simulink model "Doppelpendel_LQG_2016a"  (R2016a)
settings: Solver=ode45  StartTime=0.0  StopTime=10
values from neighbouring files (symbols this model uses):
  Beobachter_Rueckfuehrung = 0    [m8.m]
  parLQR = LQR_Entwurf( sysd,parLQR )    [m8.m]
  Quantisierung = 0    [m8.m]
undefined symbols (not defined in the file or in its folder): parDP, parKAL
libraries: cstblocks x3
settings Model: Creator=tg  LastModifiedBy=Meiner
settings DataIOCC: LimitDataPoints=on  SaveFormat=Array  SignalLoggingSaveFormat=ModelDataLogs
settings OptimizationCC: ExpressionDepthLimit=2147483647  InitFltsAndDblsToZero=on
settings DebuggingCC: UnderspecifiedInitializationDetection=Classic  MergeDetectMultiDrivingBlocksExec=none  SolverPrmCheckMsg=warning  FcnCallInpInsideContextMsg=EnableAllAsWarning  StateNameClashWarn=warning
settings HardwareCC: ProdBitPerPointer=32  ProdLargestAtomicFloat=None  ProdIntDivRoundTo=Undefined  ProdEndianess=Unspecified  ProdWordSize=32  ProdHWDeviceType=32-bit Generic
settings ModelReferenceCC: PropagateSignalLabelsOutOfModel=off
settings SFSimCC: SimParseCustomCode=off
settings GRTTargetCC: CombineOutputUpdateFcns=off  GRTInterface=on

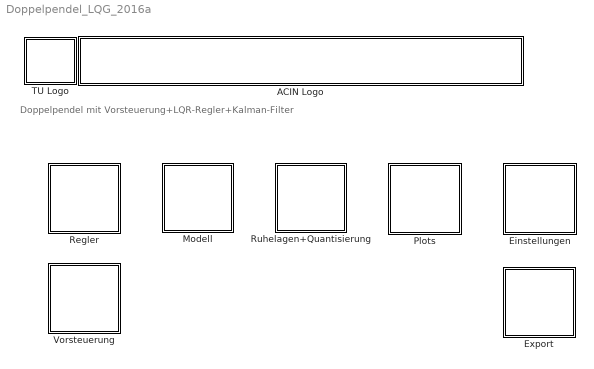
== system Doppelpendel_LQG_2016a ==
  note: Doppelpendel mit Vorsteuerung+LQR-Regler+Kalman-Filter
  ACIN Logo : Subsystem
      mask init:
      | s = get_param(gcb,'UserData');
      mask Display:
      | image(s.logo,[0 0 439 45]);
      | %axis image
  Einstellungen : Subsystem
  Export : Subsystem
  Modell : Subsystem
  Plots : Subsystem
  Regler : Subsystem
  Ruhelagen+Quantisierung : Subsystem
  TU Logo : Subsystem
      mask init:
      | s = get_param(gcb,'UserData');
      mask Display: image(s.logo,[0 0 45 45]);
  Vorsteuerung : Subsystem

== system Doppelpendel_LQG_2016a/ACIN Logo ==

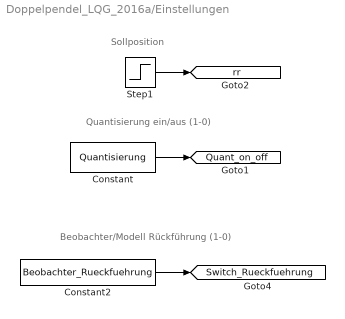
== system Doppelpendel_LQG_2016a/Einstellungen ==
  note: Sollposition
  note: Quantisierung ein/aus (1-0)
  note: Beobachter/Modell Rückführung (1-0)
  Constant : Constant  Value=Quantisierung
  Constant2 : Constant  Value=Beobachter_Rueckfuehrung
  Step1 : Step  After=0.1  SampleTime=parLQR.Ta
  tag scope: Quant_on_off=global, Switch_Rueckfuehrung=global, rr=global
  wires:
  Step1/1 -> [rr]
  Constant/1 -> [Quant_on_off]
  Constant2/1 -> [Switch_Rueckfuehrung]

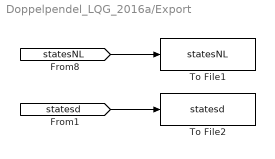
== system Doppelpendel_LQG_2016a/Export ==
  To File1 : ToFile  Filename=statesNL  MatrixName=data  SampleTime=parDP.Ta
  To File2 : ToFile  Filename=statesd  MatrixName=data  SampleTime=parDP.Ta
  wires:
  [statesNL] -> To File1/1
  [statesd] -> To File2/1

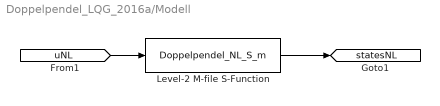
== system Doppelpendel_LQG_2016a/Modell ==
  Level-2 M-file S-Function : M-S-Function  FunctionName=Doppelpendel_NL_S_m  Parameters=parDP.phi10,parDP.omega10,parDP.phi20,parDP.omega20,parDP.s0,parDP.w0,parDP.l1,parDP.l2,parDP.a1,parDP.a2,parDP.m1,parDP.m2,parDP.J1,parDP.J2,parDP.d1,parDP.d2
  tag scope: statesNL=global
  wires:
  [uNL] -> Level-2 M-file S-Function/1
  Level-2 M-file S-Function/1 -> [statesNL]

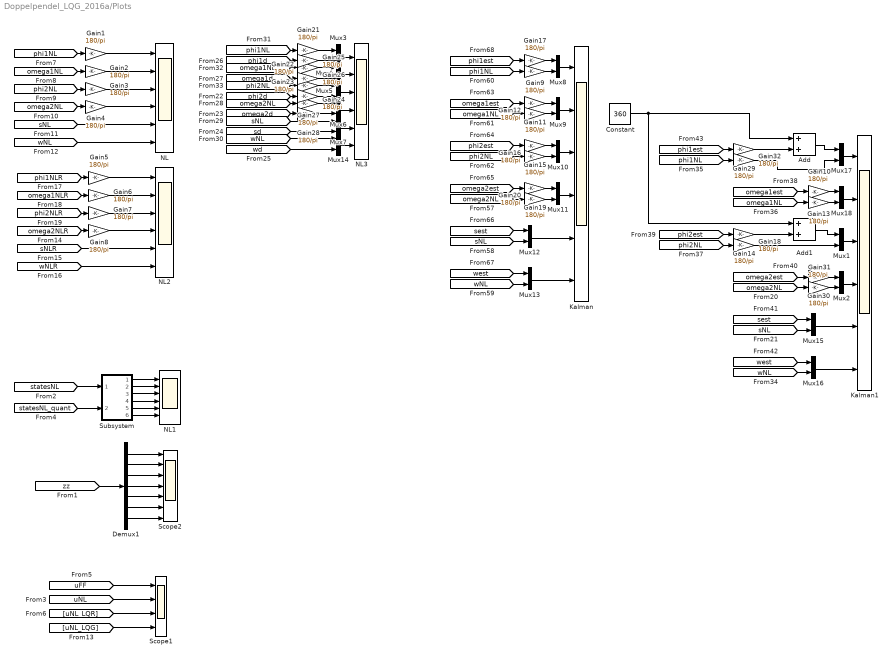
== system Doppelpendel_LQG_2016a/Plots ==
  Add : Sum
  Add1 : Sum
  Constant : Constant  Value=360
  Demux1 : Demux  Outputs=7
  Gain{1..32} (32 alike) : Gain  Gain=180/pi
  Kalman : Scope  NumInputPorts=6
  Kalman1 : Scope  NumInputPorts=6
  Mux{1..18} (18 alike) : Mux  Inputs=2
  NL{,1..3} (4 alike) : Scope  NumInputPorts=6
  Scope1 : Scope  NumInputPorts=4
  Scope2 : Scope  NumInputPorts=7
  Subsystem : Subsystem
  wires:
  [omega1NL] -> Gain2/1
  [omega2NL] -> Gain4/1
  [sNL] -> NL/5
  [wNL] -> NL/6
  Gain1/1 -> NL/1
  Gain2/1 -> NL/2
  Gain3/1 -> NL/3
  Gain4/1 -> NL/4
  [phi1NL] -> Gain1/1
  [phi2NL] -> Gain3/1
  [statesNL] -> Subsystem/1(In1)
  [statesNL_quant] -> Subsystem/2(In2)
  Subsystem/1(Out1) -> NL1/1
  Subsystem/2(Out2) -> NL1/2
  Subsystem/3(Out3) -> NL1/3
  Subsystem/4(Out4) -> NL1/4
  Subsystem/5(Out5) -> NL1/5
  Subsystem/6(Out6) -> NL1/6
  [omega1NL] -> Gain22/1
  [omega2NL] -> Gain24/1
  [phi1NL] -> Gain21/1
  [phi2NL] -> Gain23/1
  Mux3/1 -> NL3/1
  Mux4/1 -> NL3/2
  Mux5/1 -> NL3/3
  Mux6/1 -> NL3/4
  Mux7/1 -> NL3/5
  Mux14/1 -> NL3/6
  Gain21/1 -> Mux3/1
  Gain22/1 -> Mux4/1
  Gain23/1 -> Mux5/1
  Gain24/1 -> Mux6/1
  [sNL] -> Mux7/1
  [wNL] -> Mux14/1
  [phi1d] -> Gain25/1
  [omega1d] -> Gain26/1
  [phi2d] -> Gain27/1
  [omega2d] -> Gain28/1
  Gain25/1 -> Mux3/2
  Gain26/1 -> Mux4/2
  Gain27/1 -> Mux5/2
  Gain28/1 -> Mux6/2
  [sd] -> Mux7/2
  [wd] -> Mux14/2
  Demux1/1 -> Scope2/1
  Demux1/2 -> Scope2/2
  Demux1/3 -> Scope2/3
  Demux1/4 -> Scope2/4
  Demux1/5 -> Scope2/5
  Demux1/6 -> Scope2/6
  Demux1/7 -> Scope2/7
  [zz] -> Demux1/1
  Mux13/1 -> Kalman/6
  Mux12/1 -> Kalman/5
  Mux11/1 -> Kalman/4
  [omega1NL] -> Gain12/1
  [omega2NL] -> Gain20/1
  [phi1NL] -> Gain9/1
  [phi2NL] -> Gain16/1
  [sest] -> Mux12/1
  [west] -> Mux13/1
  [sNL] -> Mux12/2
  [wNL] -> Mux13/2
  Gain9/1 -> Mux8/2
  Gain17/1 -> Mux8/1
  [phi1est] -> Gain17/1
  Mux8/1 -> Kalman/1
  Gain12/1 -> Mux9/2
  Gain11/1 -> Mux9/1
  Mux9/1 -> Kalman/2
  [omega1est] -> Gain11/1
  Gain16/1 -> Mux10/2
  Gain15/1 -> Mux10/1
  [phi2est] -> Gain15/1
  Mux10/1 -> Kalman/3
  Gain20/1 -> Mux11/2
  Gain19/1 -> Mux11/1
  [omega2est] -> Gain19/1
  [uFF] -> Scope1/1
  [uNL] -> Scope1/2
  [uNL_LQR] -> Scope1/3
  [uNL_LQG] -> Scope1/4
  [omega1NLR] -> Gain6/1
  [omega2NLR] -> Gain8/1
  [sNLR] -> NL2/5
  [wNLR] -> NL2/6
  Gain5/1 -> NL2/1
  Gain6/1 -> NL2/2
  Gain7/1 -> NL2/3
  Gain8/1 -> NL2/4
  [phi1NLR] -> Gain5/1
  [phi2NLR] -> Gain7/1
  Mux16/1 -> Kalman1/6
  Mux15/1 -> Kalman1/5
  Mux2/1 -> Kalman1/4
  [omega1NL] -> Gain13/1
  [omega2NL] -> Gain31/1
  [phi1NL] -> Gain32/1
  [phi2NL] -> Gain18/1
  [sest] -> Mux15/1
  [west] -> Mux16/1
  [sNL] -> Mux15/2
  [wNL] -> Mux16/2
  Gain32/1 -> Mux17/2
  Gain29/1 -> Add/2
  [phi1est] -> Gain29/1
  Mux17/1 -> Kalman1/1
  Gain13/1 -> Mux18/2
  Gain10/1 -> Mux18/1
  Mux18/1 -> Kalman1/2
  [omega1est] -> Gain10/1
  Gain18/1 -> Mux1/2
  Gain14/1 -> Add1/2
  [phi2est] -> Gain14/1
  Mux1/1 -> Kalman1/3
  Gain31/1 -> Mux2/2
  Gain30/1 -> Mux2/1
  [omega2est] -> Gain30/1
  Add/1 -> Mux17/1
  Constant/1 -> Add/1, Add1/1
  Add1/1 -> Mux1/1

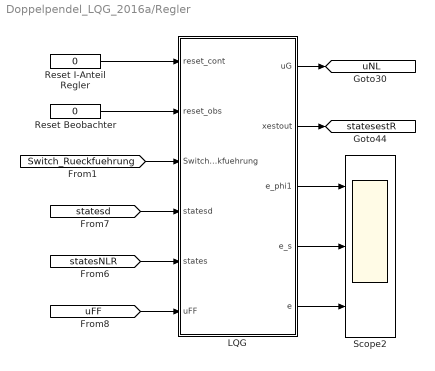
== system Doppelpendel_LQG_2016a/Regler ==
  LQG : MATLAB Function  TreatAsAtomicUnit=on
      settings: PermitHierarchicalResolution=ParametersOnly
  Reset Beobachter : Constant  Value=0
  Reset I-Anteil Regler : Constant  Value=0
  Scope2 : Scope  NumInputPorts=3
  tag scope: statesestR=global, uNL=global
  wires:
  LQG/3(e_phi1) -> Scope2/1
  LQG/4(e_s) -> Scope2/2
  LQG/5(e) -> Scope2/3
  [statesNLR] -> LQG/5(states)
  LQG/2(xestout) -> [statesestR]
  [statesd] -> LQG/4(statesd)
  [uFF] -> LQG/6(uFF)
  LQG/1(uG) -> [uNL]
  Reset Beobachter/1 -> LQG/2(reset_obs)
  Reset I-Anteil Regler/1 -> LQG/1(reset_cont)
  [Switch_Rueckfuehrung] -> LQG/3(Switch_Rueckfuehrung)

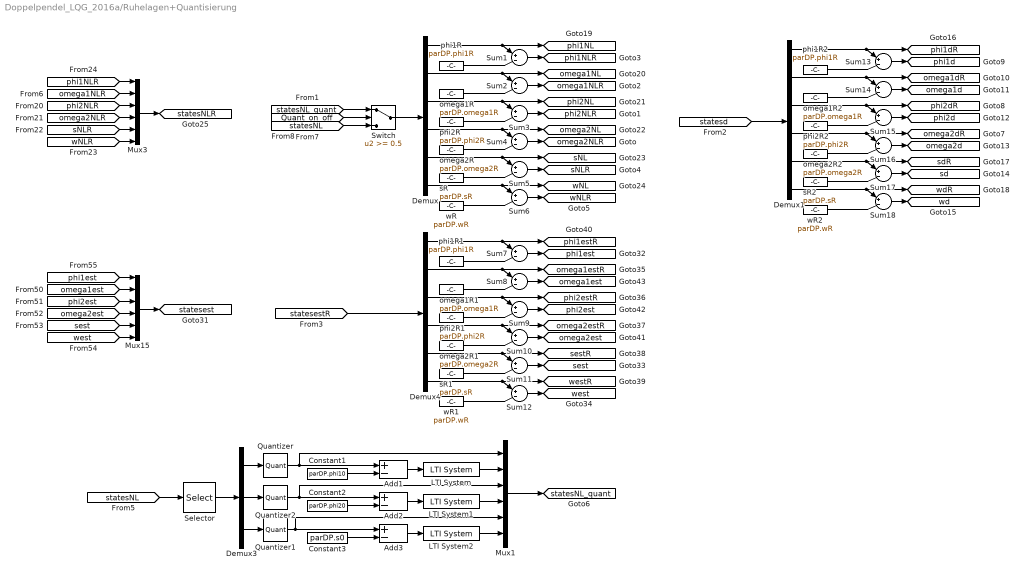
== system Doppelpendel_LQG_2016a/Ruhelagen+Quantisierung ==
  Add1 : Sum  Inputs=+-
  Add2 : Sum  Inputs=+-
  Add3 : Sum  Inputs=+-
  Constant1 : Constant  Value=parDP.phi10
  Constant2 : Constant  Value=parDP.phi20
  Constant3 : Constant  Value=parDP.s0
  Demux : Demux  Outputs=6
  Demux1 : Demux  Outputs=6
  Demux3 : Demux  Outputs=3
  Demux4 : Demux  Outputs=6
  LTI System : cstblocks/LTI System  sys=Fd_diff  IC=[]
  LTI System1 : cstblocks/LTI System  sys=Fd_diff  IC=[]
  LTI System2 : cstblocks/LTI System  sys=Fd_diff  IC=[]
  Mux1 : Mux  Inputs=6
  Mux15 : Mux  Inputs=6
  Mux3 : Mux  Inputs=6
  Quantizer : Quantizer  QuantizationInterval=Phiquantisierung  SampleTime=parLQR.Ta
  Quantizer1 : Quantizer  QuantizationInterval=Wegquantisierung  SampleTime=parLQR.Ta
  Quantizer2 : Quantizer  QuantizationInterval=Phiquantisierung  SampleTime=parLQR.Ta
  Selector : Selector  InputPortWidth=6  IndexOptions=Index vector (dialog)  Indices=[1 3 5]  OutputSizes=1
  Sum{1..18} (18 alike) : Sum  Inputs=|+-|
  Switch : Switch  Threshold=0.5
  omega1R : Constant  Value=parDP.omega1R
  omega1R1 : Constant  Value=parDP.omega1R
  omega1R2 : Constant  Value=parDP.omega1R
  omega2R : Constant  Value=parDP.omega2R
  omega2R1 : Constant  Value=parDP.omega2R
  omega2R2 : Constant  Value=parDP.omega2R
  phi1R : Constant  Value=parDP.phi1R
  phi1R1 : Constant  Value=parDP.phi1R
  phi1R2 : Constant  Value=parDP.phi1R
  phi2R : Constant  Value=parDP.phi2R
  phi2R1 : Constant  Value=parDP.phi2R
  phi2R2 : Constant  Value=parDP.phi2R
  sR : Constant  Value=parDP.sR
  sR1 : Constant  Value=parDP.sR
  sR2 : Constant  Value=parDP.sR
  wR : Constant  Value=parDP.wR
  wR1 : Constant  Value=parDP.wR
  wR2 : Constant  Value=parDP.wR
  tag scope: omega1NL=global, omega1NLR=global, omega1d=global, omega1dR=global, omega1est=global, omega1estR=global, omega2NL=global, omega2NLR=global, omega2d=global, omega2dR=global, omega2est=global, omega2estR=global, phi1NL=global, phi1NLR=global, phi1d=global, phi1dR=global, phi1est=global, phi1estR=global, phi2NL=global, phi2NLR=global, phi2d=global, phi2dR=global, phi2est=global, phi2estR=global, sNL=global, sNLR=global, sd=global, sdR=global, sest=global, sestR=global, statesNLR=global, statesNL_quant=global, statesest=global, wNL=global, wNLR=global, wd=global, wdR=global, west=global, westR=global
  wires:
  [phi1NLR] -> Mux3/1
  [omega1NLR] -> Mux3/2
  [phi2NLR] -> Mux3/3
  [omega2NLR] -> Mux3/4
  [sNLR] -> Mux3/5
  [wNLR] -> Mux3/6
  Mux3/1 -> [statesNLR]
  [phi1est] -> Mux15/1
  [omega1est] -> Mux15/2
  [phi2est] -> Mux15/3
  [omega2est] -> Mux15/4
  [sest] -> Mux15/5
  [west] -> Mux15/6
  Mux15/1 -> [statesest]
  [statesNL] -> Selector/1
  Selector/1 -> Demux3/1
  Demux3/2 -> Quantizer2/1
  Demux3/1 -> Quantizer/1
  Demux3/3 -> Quantizer1/1
  Mux1/1 -> [statesNL_quant]
  LTI System/1 -> Mux1/2
  LTI System2/1 -> Mux1/6
  LTI System1/1 -> Mux1/4
  Add1/1 -> LTI System/1
  Add2/1 -> LTI System1/1
  Add3/1 -> LTI System2/1
  Constant1/1 -> Add1/2
  Constant2/1 -> Add2/2
  Constant3/1 -> Add3/2
  Quantizer1/1 -> Add3/1, Mux1/5
  Quantizer2/1 -> Add2/1, Mux1/3
  Quantizer/1 -> Add1/1, Mux1/1
  [statesestR] -> Demux4/1
  Switch/1 -> Demux/1
  [Quant_on_off] -> Switch/2
  [statesNL_quant] -> Switch/1
  [statesNL] -> Switch/3
  [statesd] -> Demux1/1
  Sum1/1 -> [phi1NLR]
  phi1R/1 -> Sum1/2
  Demux/1 -> [phi1NL], Sum1/1
  Sum2/1 -> [omega1NLR]
  omega1R/1 -> Sum2/2
  Demux/2 -> [omega1NL], Sum2/1
  Sum3/1 -> [phi2NLR]
  phi2R/1 -> Sum3/2
  Demux/3 -> [phi2NL], Sum3/1
  Sum4/1 -> [omega2NLR]
  omega2R/1 -> Sum4/2
  Demux/4 -> [omega2NL], Sum4/1
  Sum5/1 -> [sNLR]
  sR/1 -> Sum5/2
  Demux/5 -> [sNL], Sum5/1
  Sum6/1 -> [wNLR]
  wR/1 -> Sum6/2
  Demux/6 -> [wNL], Sum6/1
  Sum7/1 -> [phi1est]
  phi1R1/1 -> Sum7/2
  Demux4/1 -> [phi1estR], Sum7/1
  Sum8/1 -> [omega1est]
  omega1R1/1 -> Sum8/2
  Demux4/2 -> [omega1estR], Sum8/1
  Sum9/1 -> [phi2est]
  phi2R1/1 -> Sum9/2
  Demux4/3 -> [phi2estR], Sum9/1
  Sum10/1 -> [omega2est]
  omega2R1/1 -> Sum10/2
  Demux4/4 -> [omega2estR], Sum10/1
  Sum11/1 -> [sest]
  sR1/1 -> Sum11/2
  Demux4/5 -> [sestR], Sum11/1
  Sum12/1 -> [west]
  wR1/1 -> Sum12/2
  Demux4/6 -> [westR], Sum12/1
  Sum13/1 -> [phi1d]
  phi1R2/1 -> Sum13/2
  Demux1/1 -> [phi1dR], Sum13/1
  Sum14/1 -> [omega1d]
  omega1R2/1 -> Sum14/2
  Demux1/2 -> [omega1dR], Sum14/1
  Sum15/1 -> [phi2d]
  phi2R2/1 -> Sum15/2
  Demux1/3 -> [phi2dR], Sum15/1
  Sum16/1 -> [omega2d]
  omega2R2/1 -> Sum16/2
  Demux1/4 -> [omega2dR], Sum16/1
  Sum17/1 -> [sd]
  sR2/1 -> Sum17/2
  Demux1/5 -> [sdR], Sum17/1
  Sum18/1 -> [wd]
  wR2/1 -> Sum18/2
  Demux1/6 -> [wdR], Sum18/1

== system Doppelpendel_LQG_2016a/TU Logo ==

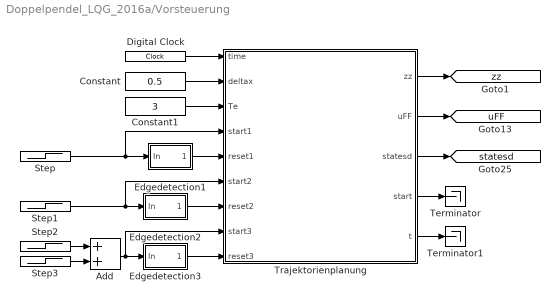
== system Doppelpendel_LQG_2016a/Vorsteuerung ==
  Add : Sum
  Constant : Constant  Value=0.5
  Constant1 : Constant  Value=3
  Digital Clock : DigitalClock  SampleTime=parLQR.Ta
  Edgedetection1 : Subsystem
  Edgedetection2 : Subsystem
  Edgedetection3 : Subsystem
  Step : Step  Time=2  SampleTime=0
  Step1 : Step  Time=6  SampleTime=0
  Step2 : Step  Time=14  After=-1  SampleTime=0
  Step3 : Step  Time=10  SampleTime=0
  Terminator : Terminator
  Terminator1 : Terminator
  Trajektorienplanung : MATLAB Function  TreatAsAtomicUnit=on
      settings: PermitHierarchicalResolution=ParametersOnly
  tag scope: statesd=global, uFF=global, zz=global
  wires:
  Trajektorienplanung/1(zz) -> [zz]
  Trajektorienplanung/5(t) -> Terminator1/1
  Trajektorienplanung/4(start) -> Terminator/1
  Step3/1 -> Add/2
  Step2/1 -> Add/1
  Edgedetection3/1(Out1) -> Trajektorienplanung/9(reset3)
  Step1/1 -> Edgedetection2/1(In), Trajektorienplanung/6(start2)
  Edgedetection2/1(Out1) -> Trajektorienplanung/7(reset2)
  Edgedetection1/1(Out1) -> Trajektorienplanung/5(reset1)
  Digital Clock/1 -> Trajektorienplanung/1(time)
  Trajektorienplanung/3(statesd) -> [statesd]
  Step/1 -> Edgedetection1/1(In), Trajektorienplanung/4(start1)
  Trajektorienplanung/2(uFF) -> [uFF]
  Constant/1 -> Trajektorienplanung/2(deltax)
  Constant1/1 -> Trajektorienplanung/3(Te)
  Add/1 -> Edgedetection3/1(In), Trajektorienplanung/8(start3)

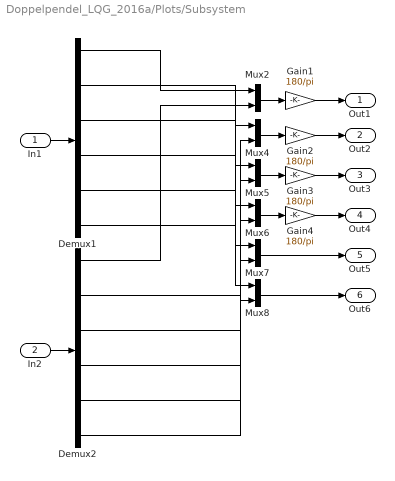
== system Doppelpendel_LQG_2016a/Plots/Subsystem ==
  In1 : Inport
  In2 : Inport  Port=2
  Demux1 : Demux  Outputs=6
  Demux2 : Demux  Outputs=6
  Gain{1..4} (4 alike) : Gain  Gain=180/pi
  Mux{2,4..8} (6 alike) : Mux  Inputs=2
  Out1 : Outport
  Out2 : Outport  Port=2
  Out3 : Outport  Port=3
  Out4 : Outport  Port=4
  Out5 : Outport  Port=5
  Out6 : Outport  Port=6
  wires:
  Demux1/1 -> Mux2/1
  Demux2/1 -> Mux2/2
  Demux2/2 -> Mux4/2
  Demux2/3 -> Mux5/2
  Demux2/4 -> Mux6/2
  Demux2/5 -> Mux7/2
  Demux2/6 -> Mux8/2
  Demux1/6 -> Mux8/1
  Demux1/5 -> Mux7/1
  Demux1/2 -> Mux4/1
  Demux1/3 -> Mux5/1
  Demux1/4 -> Mux6/1
  Mux2/1 -> Gain1/1
  Mux4/1 -> Gain2/1
  In1/1 -> Demux1/1
  Mux5/1 -> Gain3/1
  Mux6/1 -> Gain4/1
  Mux7/1 -> Out5/1
  Mux8/1 -> Out6/1
  In2/1 -> Demux2/1
  Gain1/1 -> Out1/1
  Gain2/1 -> Out2/1
  Gain3/1 -> Out3/1
  Gain4/1 -> Out4/1

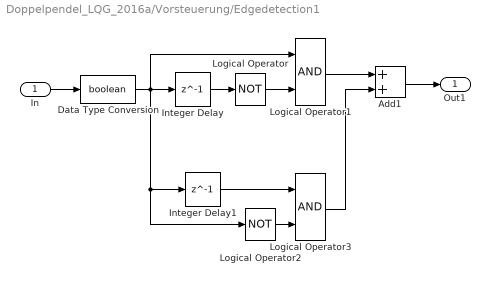
== system Doppelpendel_LQG_2016a/Vorsteuerung/Edgedetection1 ==
  In : Inport
  Add1 : Sum
  Data Type Conversion : DataTypeConversion  OutDataTypeStr=boolean  SaturateOnIntegerOverflow=on  RndMeth=Zero
  Integer Delay : Delay  DelayLength=1  InputProcessing=Inherited  SampleTime=parLQR.Ta
  Integer Delay1 : Delay  DelayLength=1  InputProcessing=Inherited  SampleTime=parLQR.Ta
  Logical Operator : Logic  Operator=NOT  Inputs=1
  Logical Operator1 : Logic
  Logical Operator2 : Logic  Operator=NOT  Inputs=1
  Logical Operator3 : Logic
  Out1 : Outport
  wires:
  In/1 -> Data Type Conversion/1
  Integer Delay/1 -> Logical Operator/1
  Data Type Conversion/1 -> Logical Operator1/1, Integer Delay/1, Integer Delay1/1, Logical Operator2/1
  Logical Operator/1 -> Logical Operator1/2
  Logical Operator2/1 -> Logical Operator3/2
  Integer Delay1/1 -> Logical Operator3/1
  Logical Operator1/1 -> Add1/1
  Logical Operator3/1 -> Add1/2
  Add1/1 -> Out1/1

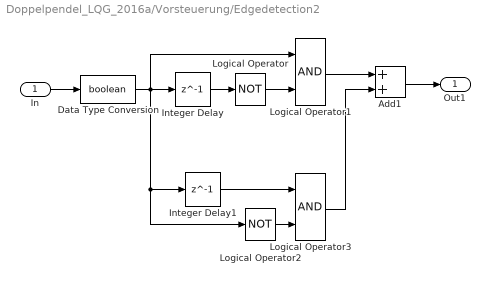
== system Doppelpendel_LQG_2016a/Vorsteuerung/Edgedetection2 ==
  In : Inport
  Add1 : Sum
  Data Type Conversion : DataTypeConversion  OutDataTypeStr=boolean  SaturateOnIntegerOverflow=on  RndMeth=Zero
  Integer Delay : Delay  DelayLength=1  InputProcessing=Inherited  SampleTime=parLQR.Ta
  Integer Delay1 : Delay  DelayLength=1  InputProcessing=Inherited  SampleTime=parLQR.Ta
  Logical Operator : Logic  Operator=NOT  Inputs=1
  Logical Operator1 : Logic
  Logical Operator2 : Logic  Operator=NOT  Inputs=1
  Logical Operator3 : Logic
  Out1 : Outport
  wires:
  Add1/1 -> Out1/1
  Logical Operator3/1 -> Add1/2
  Logical Operator1/1 -> Add1/1
  Integer Delay1/1 -> Logical Operator3/1
  Logical Operator2/1 -> Logical Operator3/2
  Logical Operator/1 -> Logical Operator1/2
  Data Type Conversion/1 -> Logical Operator2/1, Integer Delay1/1, Integer Delay/1, Logical Operator1/1
  Integer Delay/1 -> Logical Operator/1
  In/1 -> Data Type Conversion/1

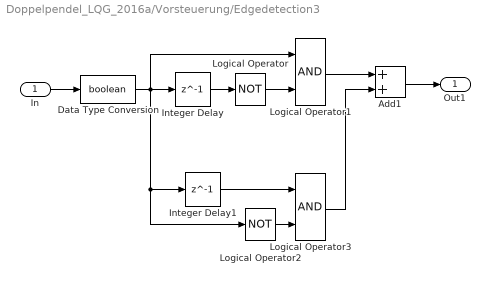
== system Doppelpendel_LQG_2016a/Vorsteuerung/Edgedetection3 ==
  In : Inport
  Add1 : Sum
  Data Type Conversion : DataTypeConversion  OutDataTypeStr=boolean  SaturateOnIntegerOverflow=on  RndMeth=Zero
  Integer Delay : Delay  DelayLength=1  InputProcessing=Inherited  SampleTime=parLQR.Ta
  Integer Delay1 : Delay  DelayLength=1  InputProcessing=Inherited  SampleTime=parLQR.Ta
  Logical Operator : Logic  Operator=NOT  Inputs=1
  Logical Operator1 : Logic
  Logical Operator2 : Logic  Operator=NOT  Inputs=1
  Logical Operator3 : Logic
  Out1 : Outport
  wires:
  In/1 -> Data Type Conversion/1
  Integer Delay/1 -> Logical Operator/1
  Data Type Conversion/1 -> Logical Operator1/1, Integer Delay/1, Integer Delay1/1, Logical Operator2/1
  Logical Operator/1 -> Logical Operator1/2
  Logical Operator2/1 -> Logical Operator3/2
  Integer Delay1/1 -> Logical Operator3/1
  Logical Operator1/1 -> Add1/1
  Logical Operator3/1 -> Add1/2
  Add1/1 -> Out1/1

== matlab function Doppelpendel_LQG_2016a/Regler/LQG ==
  settings: updateMethod=DISCRETE  sampleTime=parLQR.Ta
  data: reset_cont input; reset_obs input; Switch_Rueckfuehrung input; statesd input; states input; uFF input; uG output; parLQR parameter; xestout output; e_phi1 output; e_s output; parKAL parameter; e output
function [uG,xestout,e_phi1,e_s,e]  = LQG(reset_cont,reset_obs,Switch_Rueckfuehrung,statesd,states,uFF,parLQR,parKAL)

%Anfangsbedinungen
persistent xI
if isempty(xI) xI = double(0); end

persistent phi1est
if isempty(phi1est)phi1est = 0; end
persistent omega1est
if isempty(omega1est)omega1est = 0; end
persistent phi2est
if isempty(phi2est)phi2est = 0; end
persistent omega2est
if isempty(omega2est)omega2est = 0; end
persistent sest
if isempty(sest)sest = 0; end
persistent west
if isempty(west)west = 0; end

%Ausgang
xestout=[phi1est,omega1est,phi2est,omega2est,sest,west]';

%Beobachterrückführung ein/aus
if (Switch_Rueckfuehrung)
    xest=xestout;
else
    xest=states;
end
%%%%%%%%%%%%%%%%%%%%%%%%%%%%%%%%%%%%%%%%%%%%%%%%%%%%%%%%%%%%%%%%%%%%%%%%%%%
%LQR-Regler
%%%%%%%%%%%%%%%%%%%%%%%%%%%%%%%%%%%%%%%%%%%%%%%%%%%%%%%%%%%%%%%%%%%%%%%%%%%

% Folgendes hier bitte ausführen:
% 1.) PI-Zustandsregler einfügen

% xI(k+1) = xI(k) + (yd - y) (xI = eI)
xI = xI + (statesd(5) - xest(5));


% 2.) if (reset_cont==1) xI=0 end
if (reset_cont==1) 
    xI=0;
end

%Gesamtrückführung
% uFB = [kxT kI] [delta_e; delta_eI] (2.26b)
uG = parLQR.kx*(xest - statesd) + parLQR.kI * xI + uFF;

%%%%%%%%%%%%%%%%%%%%%%%%%%%%%%%%%%%%%%%%%%%%%%%%%%%%%%%%%%%%%%%%%%%%%%%%%%%
%Kalman-Filter
%%%%%%%%%%%%%%%%%%%%%%%%%%%%%%%%%%%%%%%%%%%%%%%%%%%%%%%%%%%%%%%%%%%%%%%%%%%

% Folgendes hier bitte ausführen:
% 1.) Kalman-Filter einfügen

xest = parKAL.Asysd*xest + parKAL.bsysd*uG + ...
    parKAL.KK*([states(5); states(1)] - [ xest(5); xest(1)]);

phi1est = xest(1);
omega1est = xest(2);
phi2est = xest(3);
omega2est = xest(4);
sest = xest(5);
west = xest(6);

% Fehler:
e_phi1 = phi1est - states(1);
e_s = sest - states(5);
e = 0;

% 2.) if (reset_obs==1) xestout=[0,0,0,0,0,0]' end
if (reset_obs==1) 
    xestout = [0,0,0,0,0,0]';
end

== matlab function Doppelpendel_LQG_2016a/Vorsteuerung/Trajektorienplanung ==
  settings: updateMethod=DISCRETE  sampleTime=parLQR.Ta
  data: time input; deltax input; Te input; zz output; parFF parameter; uFF output; statesd output; start1 input; reset1 input; start2 input; start output; reset2 input; t output; start3 input; reset3 input
%%%%%%%%%%%%%%%%%%%%%%%%%%%%%%%%%%%%%%%%%%%%%%%%%%%%%%%%%%%%%%%%%%%%%%%%%%%
%
% Trajektorienplanung zum Versetzten des Doppelpendels
%
%%%%%%%%%%%%%%%%%%%%%%%%%%%%%%%%%%%%%%%%%%%%%%%%%%%%%%%%%%%%%%%%%%%%%%%%%%%

function [zz,uFF,statesd,start,t] = Trajektorienplanung(time,deltax,Te,parFF,start1,reset1,start2,reset2,start3,reset3)

persistent tstart
if isempty(tstart) tstart = double(0); end
persistent x0
if isempty(x0) x0 = double(0); end
persistent xT
if isempty(xT) xT = double(deltax); end


if reset1>0.5 || reset2>0.5 || reset3>0.5
    
    tstart = time;

end
%Zeit ab tstart
t = time - tstart;


if  start1>0.5 
    
    start = 1;
    
    if start2<0.5
        
        x0=0;
        xT=deltax; 
        
    else
        
        if start3<0.5
        
            x0=deltax;
            xT=-deltax; 
        
        else
    
            %Anfangs- und Endwert
            x0=-deltax;
            xT=deltax;
            
        end

    end
    
else
    
    start = 0;
    
end

% Folgendes hier bitte ausführen:
% 1.) Umrechnung auf Anfangs- und Endwert des Flachen Ausgangs
% 2.) Funktion Trajektorie() ergänzen
% 3.) Vorsteuerungsberechnung uFF ergänzen
% 4.) Sollzustandsverlauf statesd ergänzen

%p Umrechnung auf Anfangs- und Endwert des Flachen Ausgangs
% parFF.VV = inv(parFF.VVinv);

z0 = parFF.VV(1,5) * x0;
zT = parFF.VV(1,5) * xT;

zz = Trajektorie(start,t,Te,z0,zT,parFF);
%zz=[z,zdot,z2dot,z3dot,z4dot,z5dot,z6dot];

%p Vorsteuerung laut S.27/(2.22)
%p zz (Delta_z) muss zu einem Spaltenvektor gemacht werden
uFF = parFF.aa'*zz';
%p Sollzustandsverlauf
statesd = parFF.VVinv*zz(1:6)';

end

%%%%%%%%%%%%%%%%%%%%%%%%%%%%%%%%%%%%%%%%%%%%%%%%%%%%%%%%%%%%%%%%%%%%%%%%%%    
function [zz] = Trajektorie(start,t,Te,z0,zT,parFF)
    
    if start<0.5

        z     = z0; 
        zdot  = 0; 
        z2dot = 0; 
        z3dot = 0; 
        z4dot = 0; 
        z5dot = 0; 
        z6dot = 0; 

    elseif start>0.5 && t<Te

        % Folgendes hier bitte ausführen:
        % 1.) Berechnung der Solltrajektorie
        beta7 = parFF.beta7/Te^7;
        beta8 = parFF.beta8/Te^8;
        beta9 = parFF.beta9/Te^9;
        beta10 = parFF.beta10/Te^10;
        beta11 = parFF.beta11/Te^11;
        beta12 = parFF.beta12/Te^12;
        beta13 = parFF.beta13/Te^13;
        
        zT_z0 = zT - z0;      
                
        z = z0 + zT_z0 * (beta7 * t.^ 7 + beta8 * t.^ 8 + beta9 * t.^ 9 + beta10 * t.^ 10 + beta11 * t.^ 11 + beta12 * t.^ 12 + beta13 * t.^ 13);
        zdot =  zT_z0 * (7 * beta7 * t.^ 6 + 8 * beta8 * t.^ 7 + 9 * beta9 * t.^ 8 + 10 * beta10 * t.^ 9 + 11 * beta11 * t.^ 10 + 12 * beta12 * t.^ 11 + 13 * beta13 * t.^ 12);
        z2dot = zT_z0 * (42 * beta7 * t.^ 5 + 56 * beta8 * t.^ 6 + 72 * beta9 * t.^ 7 + 90 * beta10 * t.^ 8 + 110 * beta11 * t.^ 9 + 132 * beta12 * t.^ 10 + 156 * beta13 * t.^ 11);
        z3dot = zT_z0 * (210 * beta7 * t.^ 4 + 336 * beta8 * t.^ 5 + 504 * beta9 * t.^ 6 + 720 * beta10 * t.^ 7 + 990 * beta11 * t.^ 8 + 1320 * beta12 * t.^ 9 + 1716 * beta13 * t.^ 10);
        z4dot = zT_z0 * (840 * beta7 * t.^ 3 + 1680 * beta8 * t.^ 4 + 3024 * beta9 * t.^ 5 + 5040 * beta10 * t.^ 6 + 7920 * beta11 * t.^ 7 + 11880 * beta12 * t.^ 8 + 17160 * beta13 * t.^ 9);
        z5dot = zT_z0 * (2520 * beta7 * t.^ 2 + 6720 * beta8 * t.^ 3 + 15120 * beta9 * t.^ 4 + 30240 * beta10 * t.^ 5 + 55440 * beta11 * t.^ 6 + 95040 * beta12 * t.^ 7 + 154440 * beta13 * t.^ 8);
        z6dot = zT_z0 * (5040 * beta7 * t + 20160 * beta8 * t.^ 2 + 60480 * beta9 * t.^ 3 + 151200 * beta10 * t.^ 4 + 332640 * beta11 * t.^ 5 + 665280 * beta12 * t.^ 6 + 1235520 * beta13 * t.^ 7);


    else

        z     = zT; 
        zdot  = 0; 
        z2dot = 0; 
        z3dot = 0; 
        z4dot = 0; 
        z5dot = 0; 
        z6dot = 0; 

    end

    zz=[z,zdot,z2dot,z3dot,z4dot,z5dot,z6dot];

end
